simulink model "ame532Project1_GimbalDynamicsModel_2022b"  (R2022b)
settings: Solver=ode4  StartTime=0.0  StopTime=10  FixedStep=0.01  RelTol=1e-3
model workspace (MAT data in the model file):
  theta : Simulink.Parameter (value not decoded)
values from neighbouring files (symbols this model uses):
  a0_s2 = 0    [AeroData.m]
  a0_s3 = 0    [AeroData.m]
  a0_s4 = 0.05    [AeroData.m]
  a0_s5 = 0.05    [AeroData.m]
  CD0_s2 = 0.01    [AeroData.m]
  CD0_s3 = 0.01    [AeroData.m]
  CD0_s4 = 0.01    [AeroData.m]
  CD0_s5 = 0.01    [AeroData.m]
  CDa_s2 = 1    [AeroData.m]
  CDa_s3 = 1    [AeroData.m]
  CDa_s4 = 1    [AeroData.m]
  CDa_s5 = 1    [AeroData.m]
  CL0_s2 = 0    [AeroData.m]
  CL0_s3 = 0    [AeroData.m]
  CL0_s4 = 0.05    [AeroData.m]
  CL0_s5 = 0.05    [AeroData.m]
  CM0_s2 = 0    [AeroData.m]
  CM0_s3 = 0    [AeroData.m]
  CM0_s4 = -0.05    [AeroData.m]
  CM0_s5 = -0.05    [AeroData.m]
  CMa_s2 = 0    [AeroData.m]
  CMa_s3 = 0    [AeroData.m]
  CMa_s4 = 0    [AeroData.m]
  CMa_s5 = 0    [AeroData.m]
  e_s2 = 0.8    [AeroData.m]
  e_s3 = 0.8    [AeroData.m]
  e_s4 = 0.9    [AeroData.m]
  e_s5 = 0.9    [AeroData.m]
  i_s2 = 0    [AeroData.m]
  i_s3 = 0    [AeroData.m]
  i_s4 = 0.05    [AeroData.m]
  i_s5 = 0.05    [AeroData.m]
  Jxx = 1    [Sim_sixDOFdriverScript.m]
  Jxy = 0.    (= 0)    [Sim_sixDOFdriverScript.m]
  Jxz = 3    [Sim_sixDOFdriverScript.m]
  Jyx = 2    [Sim_sixDOFdriverScript.m]
  Jyy = 2    [Sim_sixDOFdriverScript.m]
  Jyz = 0    [Sim_sixDOFdriverScript.m]
  Jzx = Jxz    (= 3)    [Sim_sixDOFdriverScript.m]
  Jzy = Jyz    (= 0)    [Sim_sixDOFdriverScript.m]
  Jzz = 2    [Sim_sixDOFdriverScript.m]
  LL = 0.8    [Sim_sixDOFdriverScript.m]
  MM = 0.8    [Sim_sixDOFdriverScript.m]
  n_s2 = [0; 0; -1]    [AeroData.m]
  n_s3 = [0; 1; 0]    [AeroData.m]
  n_s4 = [0; 0; -1]    [AeroData.m]
  n_s5 = [0; 0; -1]    [AeroData.m]
  NN = 0.8    [Sim_sixDOFdriverScript.m]
  rEarth = 6378100    [Sim_sixDOFdriverScript.m]
  ro = 1.225    [AeroData.m]
undefined symbols (not defined in the file or in its folder): AR_s2, AR_s3, AR_s4, AR_s5, area_s2, area_s3, area_s4, area_s5, c_s2, c_s3, c_s4, c_s5, earthRadius, elevator_sA, leftaileron_sA, mixMatrixInv, rightaileron_sA, rudder_sA, totMass, x_S2_B_B, x_S3_B_B, x_S4_B_B, x_S5_B_B
libraries: simulink_extras x35, matrix_library x22, aerolibutil x8, aerolibfltsims x4, vrlib x4, aerolibtransform2 x2, sharedtransform x2, simulink x2, slpidlib x1, sharedutil x1
(part 5 of 5)

== matlab function ame532Project1_GimbalDynamicsModel_2022b/Subsystem/Equations of Motion/Aero Forces and Moments/F&M Right Wing and Servo Surface (S5)/Compute Aero Lift and Drag ==
  data: alphaLocal output; v_B_A_B input; liftSurf output; dragSurf output; AR_s5 input; i_s5 input; n_s5 input; CL0_s5 input; CD0_s5 input; CDa_s5 input; a0_s5 input; e_s5 input; ro input; area_s5 input; leftAileronControl input; leftAileronArea_uControl input
function [alphaLocal, liftSurf, dragSurf] = fcn(v_B_A_B, AR_s5, i_s5, n_s5, CL0_s5, CD0_s5, CDa_s5, a0_s5, e_s5, ro, area_s5, leftAileronControl, leftAileronArea_uControl)
% Compute the lift and drag forces at the respective surface
% arSurf -> Aspect Ratio of respective surfaace
% ro -> air density (note: varies with altitude)
% v_infSurf -> total airspeed at the surface, i.e. Velocity of body w.r.t Inertial/ECEF as
% measured in body frame (|V_B_E_B|)
% v_B_A_B -> relative airspeed, where it is typically 
% v_B_E_B - c_B_N * v_A_N_N and v_A_N_N is the velocity of air mass w.r.t. NED 
% nSurf_B -> Normal force applied at surface
% eSurf -> Oswald efficiency
% alphaLocal0 -> Minimum drag Angle of Attack
delCLsPerdelMu = 3; % ~ About 3 per radian
v_infSurf = norm(v_B_A_B);
cSurfLocAlpha = 2*pi * (AR_s5/(2+AR_s5)); % Lift coefficient at the respective surface due to the local alpha (Angle of Attack)
alphaLocal = i_s5 - asin(dot(v_B_A_B,n_s5)/norm(v_B_A_B)); % in Radians
%cSurfLift = CL0_s5 + cSurfLocAlpha * alphaLocal; % Lift coefficient of surface
cSurfLift = CL0_s5 + cSurfLocAlpha * alphaLocal + (delCLsPerdelMu)*leftAileronControl*(leftAileronArea_uControl/area_s5); % Lift coefficient of surface
cSurfDrag = CD0_s5 + CDa_s5 *(alphaLocal - a0_s5)^2 + (cSurfLift^2/(pi*e_s5*AR_s5));

liftSurf = cSurfLift * 0.5 * ro * (v_infSurf^2)*area_s5;
dragSurf = cSurfDrag * 0.5 * ro * (v_infSurf^2)*area_s5;

== matlab function ame532Project1_GimbalDynamicsModel_2022b/Subsystem/Equations of Motion/Aero Forces and Moments/F&M Right Wing and Servo Surface (S5)/Compute Aero Moment ==
  data: V_B_A_B input; momSurf output; alphaLocal input; CM0_s5 input; CMa_s5 input; ro input; area_s5 input; c_s5 input
function momSurf = fcn(V_B_A_B, alphaLocal, CM0_s5, CMa_s5, ro, area_s5, c_s5)
% Compute the Moment at the respective Surface
% v_infSurf -> total airspeed at the surface, i.e. Velocity of body w.r.t Inertial/ECEF as
% measured in body frame (|V_B_E_B|)
% ro -> air density (note: varies with altitude)
% chordSurf -> Chord of the surface area
% cSurfM0 -> Initial moment coefficient of surface
% cSurfMalpha -> Moment coefficient at the respective surface due to the
% local alpha (Angle of Attack)
v_infSurf = norm(V_B_A_B);
cSurfMom = CM0_s5 + CMa_s5*alphaLocal; % Moment coefficient of surface
momSurf = cSurfMom * 0.5 * ro * (v_infSurf^2)*area_s5 * c_s5;

== matlab function ame532Project1_GimbalDynamicsModel_2022b/Subsystem/Equations of Motion/Aero Forces and Moments/F&M Right Wing and Servo Surface (S5)/F&M in Body/Force Due to Lift and Drag ==
  data: lift input; forceLiftDragS5_B output; drag input; v_B_A_B input; n_s5 input
function forceLiftDragS5_B = fcn(lift, drag, v_B_A_B, n_s5)

forceLiftDrag_w = lift*n_s5 - [drag; 0; 0];
alpha = atan2(v_B_A_B(3), v_B_A_B(1));
beta = asin(v_B_A_B(2) / norm(v_B_A_B));

c_S_B = [cos(alpha), 0, sin(alpha); 0, 1, 0; -sin(alpha), 0, cos(alpha)] ;
c_W_S = [cos(beta), sin(beta), 0; -sin(beta), cos(beta), 0; 0,0,1];
c_W_B = c_W_S * c_S_B;

forceLiftDragS5_B = c_W_B' * forceLiftDrag_w;
